simulink model "aeropendulum_model"  (R2021b)
settings: Solver=FixedStepAuto  StartTime=0.0  StopTime=900  FixedStep=0.01  RelTol=1e-3
model workspace (MATLAB code in the model file):
  | %Dane do wahadla
  | m=0.120; %masa wahadla [kg]
  | g=9.81; %przyspieszenie grawitacyjne [m/s^2]
  | c=0.00700; %tarcie wiskotyczne [Nms/rad] https://koyo.jtekt.co.jp/en/support/bearing-knowledge/8-4000.html
  | l=0.25; %dlugosc wahadla [m]
  | J=m*l*l; %moment bezwladnosci [kgm^2] https://www.youtube.com/watch?v=scIVIhChL1I
  | d=0.25; %odleglosc osi od srodka masy https://youtu.be/2KCuR6kIrfI?t=294
  | %alfa=0.014; %wspolczynnik dla smigla w zla strone
  | %alfa_rev=0.019 %wspolczynnik dla smigla w dobra strone
libraries: simulink x1
settings Model: Creator=Barti  LastModifiedBy=adria
settings SolverCC: AlgebraicLoopSolver=TrustRegion
settings DataIOCC: ReturnWorkspaceOutputs=off
settings DebuggingCC: SFMachineParentedDataDiag=warning  ArithmeticOperatorsInVariantConditions=warning
settings SFSimCC: SimUseLocalCustomCode=off  CustomCodeUndefinedFunction=UseInterfaceOnly
settings RTWCC: RTWUseLocalCustomCode=off
settings CodeAppCC: StateflowObjectComments=on

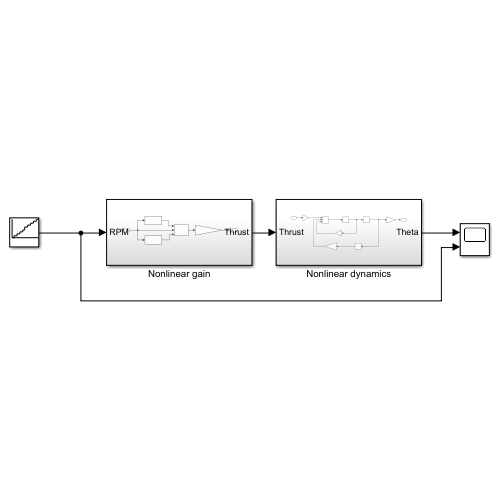
[thumbnail: Simulink's stored preview of the top-level diagram]
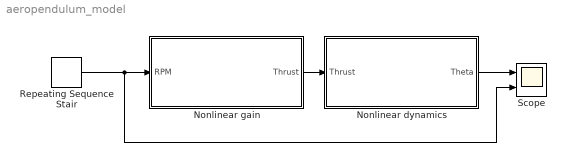
== system aeropendulum_model ==
  Nonlinear dynamics : Subsystem
  Nonlinear gain : Subsystem
  Repeating Sequence Stair : simulink/Sources/Repeating Sequence Stair  OutValues=[0 : 500 : 4500]  tsamp=10  OutMin=[]  OutMax=[]  OutDataTypeStr=double  OutputDataTypeScalingMode=double  OutDataType=fixdt(0,8)  ConRadixGroup=Best Precision: Vector-wise  OutScaling=2^-12
  Scope : Scope  NumInputPorts=2
  wires:
  Nonlinear dynamics/1(Theta) -> Scope/1
  Nonlinear gain/1(Thrust) -> Nonlinear dynamics/1(Thrust)
  Repeating Sequence Stair/1 -> Scope/2, Nonlinear gain/1(RPM)

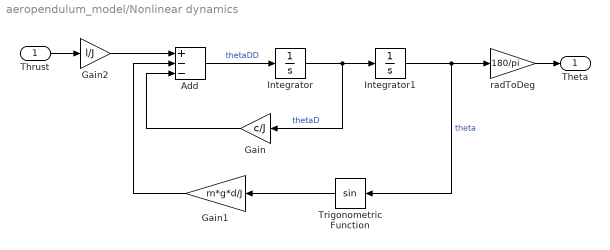
== system aeropendulum_model/Nonlinear dynamics ==
  Thrust : Inport
  Add : Sum  Inputs=+--
  Gain : Gain  Gain=c/J
  Gain1 : Gain  Gain=m*g*d/J
  Gain2 : Gain  Gain=l/J
  Integrator : Integrator
  Integrator1 : Integrator
  Trigonometric Function : Trigonometry
  radToDeg : Gain  Gain=180/pi
  Theta : Outport
  wires:
  Add/1 -> Integrator/1  "thetaDD"
  Gain2/1 -> Add/1
  Integrator/1 -> Gain/1, Integrator1/1  "thetaD"
  Gain1/1 -> Add/2
  Gain/1 -> Add/3
  Trigonometric Function/1 -> Gain1/1
  Integrator1/1 -> Trigonometric Function/1, radToDeg/1  "theta"
  Thrust/1 -> Gain2/1
  radToDeg/1 -> Theta/1

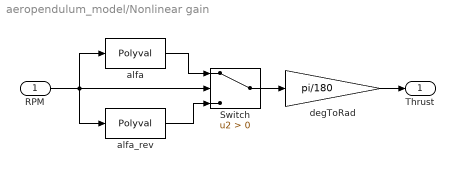
== system aeropendulum_model/Nonlinear gain ==
  RPM : Inport
  Switch : Switch  Criteria=u2 > Threshold
  alfa : Polyval  Coefs="[3.04986021927422e-06,  -0.00476887717971010 , 2.51670431281220]"
  alfa_rev : Polyval  Coefs="[-5.46944010985214e-06,\t-0.00938361577873603,\t-2.43262552689868]"
  degToRad : Gain  Gain=pi/180
  Thrust : Outport
  wires:
  RPM/1 -> alfa_rev/1, alfa/1, Switch/2
  Switch/1 -> degToRad/1
  alfa/1 -> Switch/1
  alfa_rev/1 -> Switch/3
  degToRad/1 -> Thrust/1
